simulink model "cplxfir"  (Simulink 7.4)
settings: Solver=VariableStepDiscrete  SolverMode=SingleTasking  StartTime=0.0  StopTime=.01  FixedStep=1/Fs  RelTol=1e-3
PreLoadFcn:
  | cplxfir_PreLoadFcn
values from neighbouring files (symbols this model uses):
  coefwidth = 14    [cplxfir_PreLoadFcn.m]
  Fs = 1000000    [cmplx_coef.mat]
  im_num = [0 0.000398348009628 0.00104175614283 0.00211081091276 0.00279070112666 0.00258044261419 0.000985988872345 -0.0017034426046 -0.00446098448822 -0.00593463418221 -0.00527808120455 -0.00289469541568 ... (64 elements, 1x64)]    [cmplx_coef.mat]
  re_num = [0.000255022274952 0.000745256708112 0.000696079200562 0.00020789672902 -0.00115594625519 -0.00314427842297 -0.00495690079674 -0.00561549770163 -0.00446098448822 -0.0018002515976 0.00104987562762 0.00237561513355 ... (64 elements, 1x64)]    [cmplx_coef.mat]
undefined symbols (not defined in the file or in its folder): c, C, D, d, j, sided, Two, xlipgetpartsetting
libraries: xbsIndex_r4 x23, dsparch3 x4, dspsnks4 x3, dspobslib x2, dspsrcs4 x1, xbsCopyrightNotice_r4 x1
settings Model: Creator=mklusman  LastModifiedBy=douangp
settings DataIOCC: SignalLoggingName=sigsOut
settings OptimizationCC: BooleanDataType=off  InitFltsAndDblsToZero=on
settings DebuggingCC: SaveWithParameterizedLinksMsg=none  SignalResolutionControl=TryResolveAllWithWarning  SolverPrmCheckMsg=none  MultiTaskDSMMsg=warning  MultiTaskCondExecSysMsg=none  StrictBusMsg=None
settings HardwareCC: TargetUnknown=on
settings RTWCC: IncludeERTFirstTime=on
settings GRTTargetCC: TargetFcnLib=ansi_tfl_tmw.mat

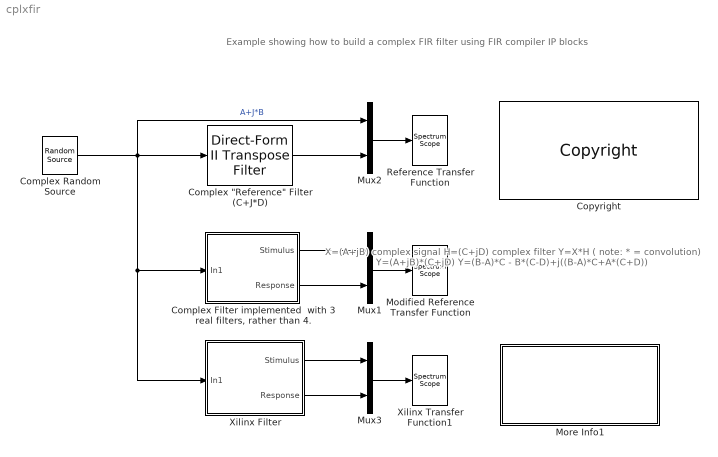
== system cplxfir ==
  note: X=(A+jB)     complex signal
      | H=(C+jD)     complex filter
      | Y=X*H ( note: * = convolution)
      | Y=(A+jB)*(C+jD)
      | Y=(B-A)*C - B*(C-D)+j((B-A)*C+A*(C+D))
  note: Example showing how to build a complex FIR filter
      |  using FIR compiler IP blocks
  "Complex \"Reference\" Filter (C+J*D)" : dsparch3/Direct-Form II Transpose Filter  num=[re_num+j*im_num]  den=1  ic=0
  "Complex Filter implemented  with 3 real filters, rather than 4.  " : Subsystem
  Complex Random Source : dspsrcs4/Random Source  SrcType=Uniform  NormMethod=Ziggurat  CltLength=12  MinVal=-.99  MaxVal=0.99  MeanVal=0  VarVal=1  RepMode=Not repeatable  rawSeed=1  IsInherit=off  SampMode=Discrete  SampTime=1/Fs  SampFrame=1  DataType=Double  OutComplex=Complex
  Copyright : xbsCopyrightNotice_r4/Copyright  copyrighttext="Copyright (c) 2010  by  Xilinx, Inc. All rights reserved.<br><br>This file contains proprietary, confidential information of Xilinx, Inc., is distributed under licensefrom Xilinx, Inc., and may be used, copied and/or disclosed only pursuant to the terms of a valid licenseagreement with Xilinx, Inc. Xilinx hereby grants you a license to use this file solely for design,simulation, implementation and creation of design files limited to Xilinx devices or technologies. Use with non-Xilinx devices or technologies is expressly prohibited and immediately terminates your license unless covered by a separate agreement.<br><br>Xilinx is providing this design, code, or information \"as-is\" solely for use in developing programs and solutions for Xilinx devices, with no obligation on the part of Xilinx to provide support. By providingthis design, code, or information as one possible implementation of this feature, application or standard,Xilinx is making no representation that this implementation is free from any claims of infringement. Youare responsible for obtaining any rights you may require for your implementation. Xilinx expressly disclaimsany warranty whatsoever with respect to the adequacy of the implementation, including but not limited to anywarranties or representations that this implementation is free from claims of infringement, implied warrantiesof merchantability or fitness for a particular purpose.<br><br>Xilinx products are not intended for use in life support appliances, devices, or systems. Use in such applications is expressly prohibited.<br><br>Any modifications that are made to the Source Code are done at the user's sole risk and will be unsupported.<br><br>This copyright and support notice must be retained as part of this text at all times. (c) Copyright 1995-2010 Xilinx, Inc. All rights reserved."  block_type=copyright
      settings: block_version=10.1.3
      settings: infoedit=|
      | Copyright(C) 2008 by  Xilinx, Inc. All rights reserved.<br>
      | <br>
      | This file contains proprietary, confidential information of Xilinx, Inc., is distributed under license
      | from Xilinx, Inc., and may be used, copied and/or disclosed only pursuant to the terms of a valid license
      | agreement with Xilinx, Inc. Xilinx hereby grants you a license to use this file solely for design,
      | simulation, implementation and creation of design files limited to Xilinx devices or technologies. Use
      | with non-Xilinx devices or technologies is expressly prohibited and immediately terminates your license
      | unless covered by a separate agreement.<br>
      | <br>
      | Xilinx is providing this design, code, or information "as-is" solely for use in developing programs and
      | solutions for Xilinx devices, with no obligation on the part of Xilinx to provide support. By providing
      | this design, code, or information as one possible implementation of this feature, application or standard,
      | Xilinx is making no representation that this implementation is free from any claims of infringement. You
      | are responsible for obtaining any rights you may require for your implementation. Xilinx expressly disclaims
      | any warranty whatsoever with respect to the adequacy of the implementation, including but not limited to any
      | warranties or representations that this implementation is free from claims of infringement, implied warranties
      | of merchantability or fitness for a particular purpose.<br>
      | <br>
      | Xilinx products are not intended for use in life support appliances, devices, or systems. Use in such
      | applications is expressly prohibited.<br>
      | <br>
      | Any modifications that are made to the Source Code are done at the user's sole risk and will be unsupported.<br>
      | <br>
      | This copyright and support notice must be retained as part of this text at all times.
      | (c) Copyright 1995-2008 Xilinx, Inc. All rights reserved.
  Modified Reference Transfer Function : dspsnks4/Spectrum Scope  DialogController=dspdialog.SpectrumScope  DialogControllerArgs=DataTag1  SystemSampleTime=-1  ScopeProperties=off  Domain=Frequency  HorizSpan=1  UseBuffer=on  BufferSize=512  Overlap=64  inpFftLenInherit=off  FFTlength=512  numAvg=2  DisplayProperties=off  AxisGrid=on  Memory=off  FrameNumber=on  AxisLegend=on  AxisZoom=off  OpenScopeAtSimStart=on  OpenScopeImmediately=off  FigPos=[-999 166 385 234]  AxisProperties=on  XUnits=Hertz  XRange=Two-sided ((-Fs/2...Fs/2])  XDisplay=0  InheritXIncr=on  XIncr=1.0  XLabel=Samples  XLimit=User-defined  YUnits=dBm  XMax=500000  XMin=0  YLabel=Magnitude, dB  LineProperties=off  LineColors=[0 0 1]|[1 0 0]  wintypeSpecScope=Hann  RsSpecScope=50  betaSpecScope=5  winsampSpecScope=Periodic  XAxisParamsVer=6.9
      settings: YMin=-91.486  YMax=10.5651
  More Info1 : Subsystem
      mask Display: disp('Double click\n for\n more information.')
  Mux1 : Mux  Inputs=2
  Mux2 : Mux  Inputs=2
  Mux3 : Mux  Inputs=2
  Reference Transfer Function : dspsnks4/Spectrum Scope  DialogController=dspdialog.SpectrumScope  DialogControllerArgs=DataTag2  SystemSampleTime=-1  ScopeProperties=off  Domain=Frequency  HorizSpan=1  UseBuffer=on  BufferSize=512  Overlap=64  inpFftLenInherit=off  FFTlength=512  numAvg=2  DisplayProperties=off  AxisGrid=on  Memory=off  FrameNumber=on  AxisLegend=on  AxisZoom=off  OpenScopeAtSimStart=on  OpenScopeImmediately=off  FigPos=[-993 480 377 230]  AxisProperties=on  XUnits=Hertz  XRange=Two-sided ((-Fs/2...Fs/2])  XDisplay=0  InheritXIncr=on  XIncr=1.0  XLabel=Samples  XLimit=User-defined  YUnits=dBm  XMax=500000  XMin=0  YLabel=Magnitude, dB  LineProperties=off  LineColors=[0 0 1]|[1 0 0]  wintypeSpecScope=Hann  RsSpecScope=50  betaSpecScope=5  winsampSpecScope=Periodic  XAxisParamsVer=6.9
      settings: YMin=-91.486  YMax=10.5651
  Xilinx Transfer Function1 : dspsnks4/Spectrum Scope  DialogController=dspdialog.SpectrumScope  DialogControllerArgs=DataTag3  SystemSampleTime=-1  ScopeProperties=off  Domain=Frequency  HorizSpan=1  UseBuffer=on  BufferSize=512  Overlap=64  inpFftLenInherit=off  FFTlength=512  numAvg=2  DisplayProperties=off  AxisGrid=on  Memory=off  FrameNumber=on  AxisLegend=on  AxisZoom=off  OpenScopeAtSimStart=on  OpenScopeImmediately=off  FigPos=[-611 244 385 234]  AxisProperties=on  XUnits=Hertz  XRange=Two-sided ((-Fs/2...Fs/2])  XDisplay=0  InheritXIncr=on  XIncr=1.0  XLabel=Samples  XLimit=User-defined  YUnits=dBm  XMax=500000  XMin=0  YLabel=Magnitude, dB  LineProperties=off  LineColors=[0 0 1]|[1 0 0]  wintypeSpecScope=Hann  RsSpecScope=50  betaSpecScope=5  winsampSpecScope=Periodic  XAxisParamsVer=6.9
      settings: YMin=-86.1357  YMax=10.4347
  Xilinx Filter : Subsystem
  wires:
  Complex Random Source/1 -> "Complex \"Reference\" Filter (C+J*D)"/1, Xilinx Filter/1(In1), "Complex Filter implemented  with 3 real filters, rather than 4.  "/1(In1), Mux2/1  "A+J*B"
  Xilinx Filter/2("Response ") -> Mux3/2
  "Complex \"Reference\" Filter (C+J*D)"/1 -> Mux2/2
  "Complex Filter implemented  with 3 real filters, rather than 4.  "/2(Response) -> Mux1/2
  Xilinx Filter/1("Stimulus ") -> Mux3/1
  Mux3/1 -> Xilinx Transfer Function1/1
  "Complex Filter implemented  with 3 real filters, rather than 4.  "/1(Stimulus) -> Mux1/1
  Mux1/1 -> Modified Reference Transfer Function/1
  Mux2/1 -> Reference Transfer Function/1

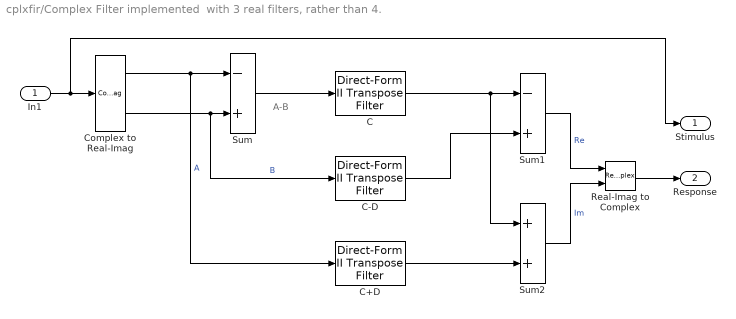
== system cplxfir/Complex Filter implemented  with 3 real filters, rather than 4.   ==
  note: A-B
  In1 : Inport  OutDataType=sfix(16)  OutScaling=2^0
  C : dsparch3/Direct-Form II Transpose Filter  num="[re_num]   %    c"  den=1  ic=0
  C+D : dsparch3/Direct-Form II Transpose Filter  num="[re_num+im_num]  % C+D"  den=1  ic=0
  C-D : dsparch3/Direct-Form II Transpose Filter  num="[re_num-im_num]    % c-d"  den=1  ic=0
  Complex to Real-Imag : ComplexToRealImag
  Real-Imag to Complex : RealImagToComplex
  Sum : Sum  Inputs=-+  OutDataType=sfix(16)  OutScaling=2^0  SaturateOnIntegerOverflow=on  InputSameDT=on  OutDataTypeStr=Inherit: Same as first input
  Sum1 : Sum  Inputs=-+  OutDataType=sfix(16)  OutScaling=2^0  SaturateOnIntegerOverflow=on  InputSameDT=on  OutDataTypeStr=Inherit: Same as first input
  Sum2 : Sum  OutDataType=sfix(16)  OutScaling=2^0  SaturateOnIntegerOverflow=on  InputSameDT=on  OutDataTypeStr=Inherit: Same as first input
  Stimulus : Outport  OutDataType=sfix(16)  OutScaling=2^0
  Response : Outport  Port=2  OutDataType=sfix(16)  OutScaling=2^0
  wires:
  Complex to Real-Imag/1 -> Sum/1, C+D/1  "A"
  Complex to Real-Imag/2 -> Sum/2, C-D/1  "B"
  Sum/1 -> C/1
  C/1 -> Sum1/1, Sum2/1
  C-D/1 -> Sum1/2
  C+D/1 -> Sum2/2
  Sum1/1 -> Real-Imag to Complex/1  "Re"
  Sum2/1 -> Real-Imag to Complex/2  "Im"
  In1/1 -> Complex to Real-Imag/1, Stimulus/1
  Real-Imag to Complex/1 -> Response/1

== system cplxfir/More Info1 ==
  note: This design shows how to migrate a complex filter design from using DAFIR to FIR
      | Compiler. The model was originally constructed using DAFIR as provided
      | by System Generator design example.   The migration process is seamless and
      | straight forward.
      |
      | The "cplxfir_PreLoadFcn.m" file is preloaded when opening the model. It also loads
      | filter coefficients stored in "cmplx_coef.mat" file. Out of the box, the model can be
      | simulated and compared between Xilinx transfer function, simulation results and
      | two other models.
      |
      | The following quality of results (QoR) are used as a reference, baseline only and they may be
      | varied within an acceptable range from one release to the next.
      | This design occupies 274 Slice LUTs, 486 Slice Registers, and 192 dedicated multipliers of
      | a Xilinx xc6vsx315t-1 part and operates close to 350 MHz (11.2 software, VHDL synthesized with
      | XST). The QoR may be further improved in both area utilizations and speed.
  note: Example showing how to build a complex FIR filter
      |  using FIR compiler IP blocks

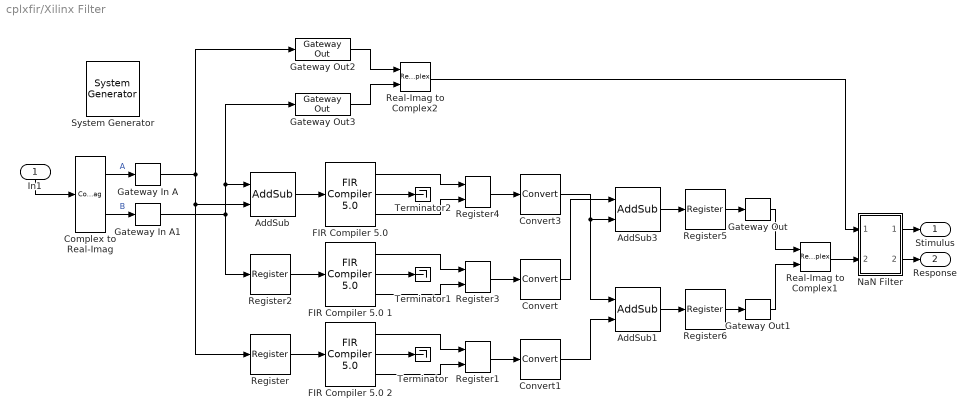
== system cplxfir/Xilinx Filter ==
  In1 : Inport  OutDataType=sfix(16)  OutScaling=2^0
  " System Generator" : xbsIndex_r4/ System Generator  Tag=genX  SystemSampleTime=-1  xilinxfamily=virtex6  part=xc6vsx315t  speed=-1  package=ff1156  synthesis_tool=XST  clock_wrapper=Clock Enables  directory=./timing  testbench=off  simulink_period=1/1000000  sysclk_period=10  dcm_input_clock_period=5  incr_netlist=off  trim_vbits=According to Block Masks  dbl_ovrd=According to Block Masks  core_generation=According to Block Masks  run_coregen=off  deprecated_control=off  eval_field=0  block_type=sysgen
      settings: block_version=9.1.01
  AddSub : xbsIndex_r4/AddSub  mode=Subtraction  use_carryin=off  use_carryout=off  en=off  latency=1  precision=Full  arith_type=Unsigned  n_bits=8  bin_pt=2  quantization=Truncate  overflow=Wrap  dbl_ovrd=off  use_behavioral_HDL=on  hw_selection=Fabric  pipelined=off  use_rpm=off  block_type=addsub
      settings: xl_area=[0, 0, 0, 0, 0, 0, 0]  block_version=VER_STRING_GOES_HERE
  AddSub1 : xbsIndex_r4/AddSub  mode=Addition  use_carryin=off  use_carryout=off  en=off  latency=1  precision=Full  arith_type=Unsigned  n_bits=8  bin_pt=2  quantization=Truncate  overflow=Wrap  dbl_ovrd=off  use_behavioral_HDL=on  hw_selection=Fabric  pipelined=off  use_rpm=off  block_type=addsub
      settings: xl_area=[0, 0, 0, 0, 0, 0, 0]  block_version=VER_STRING_GOES_HERE
  AddSub3 : xbsIndex_r4/AddSub  mode=Subtraction  use_carryin=off  use_carryout=off  en=off  latency=1  precision=Full  arith_type=Unsigned  n_bits=8  bin_pt=2  quantization=Truncate  overflow=Wrap  dbl_ovrd=off  use_behavioral_HDL=on  hw_selection=Fabric  pipelined=off  use_rpm=off  block_type=addsub
      settings: xl_area=[0, 0, 0, 0, 0, 0, 0]  block_version=VER_STRING_GOES_HERE
  Complex to Real-Imag : ComplexToRealImag
  Convert : xbsIndex_r4/Convert  arith_type="Signed  (2's comp)"  n_bits=coefwidth  bin_pt=coefwidth-2  quantization=Truncate  overflow=Wrap  en=off  latency=0  dbl_ovrd=off  pipeline=off  block_type=convert
      settings: infoedit=The input is presented at the output after quantization and overflow effects.<P><P>Hardware notes: Additional hardware is used when rounding or saturation is selected and output width is less than the input width.  xl_area=[0, 0, 0, 0, 0, 0, 0]  block_version=VER_STRING_GOES_HERE
  Convert1 : xbsIndex_r4/Convert  arith_type="Signed  (2's comp)"  n_bits=coefwidth  bin_pt=coefwidth-2  quantization=Truncate  overflow=Wrap  en=off  latency=0  dbl_ovrd=off  pipeline=off  block_type=convert
      settings: infoedit=The input is presented at the output after quantization and overflow effects.<P><P>Hardware notes: Additional hardware is used when rounding or saturation is selected and output width is less than the input width.  xl_area=[0, 0, 0, 0, 0, 0, 0]  block_version=VER_STRING_GOES_HERE
  Convert3 : xbsIndex_r4/Convert  arith_type="Signed  (2's comp)"  n_bits=coefwidth  bin_pt=coefwidth-2  quantization=Truncate  overflow=Wrap  en=off  latency=0  dbl_ovrd=off  pipeline=off  block_type=convert
      settings: infoedit=The input is presented at the output after quantization and overflow effects.<P><P>Hardware notes: Additional hardware is used when rounding or saturation is selected and output width is less than the input width.  xl_area=[0, 0, 0, 0, 0, 0, 0]  block_version=VER_STRING_GOES_HERE
  "FIR Compiler 5.0 " : xbsIndex_r4/FIR Compiler 5.0   coefficientvector=re_num  coefficient_sets=1  filter_type=Single_Rate  rate_change_type=Integer  interpolation_rate=1  decimation_rate=1  zero_pack_factor=1  number_channels=1  ratespecification=Maximum_Possible  sampleperiod=1  hardwareoversamplingrate=1  filter_architecture=Transpose_Multiply_Accumulate  coefficient_reload=off  coefficient_structure=Non_Symmetric  coefficient_sign=Signed  quantization=Quantize_Only  coefficient_width=14  bestprecision=on  coefficient_fractional_bits=6  number_paths=1  output_rounding_mode=Full_Precision  output_width=30  allow_rounding_approximation=off  optimization_goal=Speed  has_sclr=off  has_data_valid=off  has_nd=off  has_ce=off  usechan_in_adv=off  chan_in_adv=0  data_buffer_type=Automatic  coefficient_buffer_type=Automatic  input_buffer_type=Automatic  output_buffer_type=Automatic  preference_for_other_storage=Automatic  multi_column_support=Disabled  columnconfig='1'  inter_column_pipe_length=4  passband_min=0.0  passband_max=0.5  stopband_min=0.5  stopband_max=1.0  filter_selection=1  gui_behaviour=Sysgen  registered_output=true  data_sign=Signed  data_width=16  wrapper_available=true  ip_wrap_arbitrary_binary_point=true  ip_name=FIR Compiler  ip_version=5.0  dsptool_ready=true  ipcore_usecache=true  ipcore_useipmodelcache=true  ipcore_xco_need_fpga_part=true  port_translation_map={ 'ce' => 'en', 'sclr' => 'rst' }  run_core_at_system_period=true  ipcore_fpga_part=xlipgetpartsetting(gcb, {'virtex4', 'xc4vsx35', '-10', 'ff668'})  structural_sim=false  block_type=fir_compiler_v5_0
      settings: block_version=11.2
  FIR Compiler 5.0 1 : xbsIndex_r4/FIR Compiler 5.0   coefficientvector=re_num  coefficient_sets=1  filter_type=Single_Rate  rate_change_type=Integer  interpolation_rate=1  decimation_rate=1  zero_pack_factor=1  number_channels=1  ratespecification=Maximum_Possible  sampleperiod=1  hardwareoversamplingrate=1  filter_architecture=Transpose_Multiply_Accumulate  coefficient_reload=off  coefficient_structure=Non_Symmetric  coefficient_sign=Signed  quantization=Quantize_Only  coefficient_width=14  bestprecision=on  coefficient_fractional_bits=6  number_paths=1  output_rounding_mode=Full_Precision  output_width=30  allow_rounding_approximation=off  optimization_goal=Speed  has_sclr=off  has_data_valid=off  has_nd=off  has_ce=off  usechan_in_adv=off  chan_in_adv=0  data_buffer_type=Automatic  coefficient_buffer_type=Automatic  input_buffer_type=Automatic  output_buffer_type=Automatic  preference_for_other_storage=Automatic  multi_column_support=Disabled  columnconfig='1'  inter_column_pipe_length=4  passband_min=0.0  passband_max=0.5  stopband_min=0.5  stopband_max=1.0  filter_selection=1  gui_behaviour=Sysgen  registered_output=true  data_sign=Signed  data_width=16  wrapper_available=true  ip_wrap_arbitrary_binary_point=true  ip_name=FIR Compiler  ip_version=5.0  dsptool_ready=true  ipcore_usecache=true  ipcore_useipmodelcache=true  ipcore_xco_need_fpga_part=true  port_translation_map={ 'ce' => 'en', 'sclr' => 'rst' }  run_core_at_system_period=true  ipcore_fpga_part=xlipgetpartsetting(gcb, {'virtex4', 'xc4vsx35', '-10', 'ff668'})  structural_sim=false  block_type=fir_compiler_v5_0
      settings: block_version=11.2
  FIR Compiler 5.0 2 : xbsIndex_r4/FIR Compiler 5.0   coefficientvector=re_num  coefficient_sets=1  filter_type=Single_Rate  rate_change_type=Integer  interpolation_rate=1  decimation_rate=1  zero_pack_factor=1  number_channels=1  ratespecification=Maximum_Possible  sampleperiod=1  hardwareoversamplingrate=1  filter_architecture=Transpose_Multiply_Accumulate  coefficient_reload=off  coefficient_structure=Non_Symmetric  coefficient_sign=Signed  quantization=Quantize_Only  coefficient_width=14  bestprecision=on  coefficient_fractional_bits=6  number_paths=1  output_rounding_mode=Full_Precision  output_width=30  allow_rounding_approximation=off  optimization_goal=Speed  has_sclr=off  has_data_valid=off  has_nd=off  has_ce=off  usechan_in_adv=off  chan_in_adv=0  data_buffer_type=Automatic  coefficient_buffer_type=Automatic  input_buffer_type=Automatic  output_buffer_type=Automatic  preference_for_other_storage=Automatic  multi_column_support=Disabled  columnconfig='1'  inter_column_pipe_length=4  passband_min=0.0  passband_max=0.5  stopband_min=0.5  stopband_max=1.0  filter_selection=1  gui_behaviour=Sysgen  registered_output=true  data_sign=Signed  data_width=16  wrapper_available=true  ip_wrap_arbitrary_binary_point=true  ip_name=FIR Compiler  ip_version=5.0  dsptool_ready=true  ipcore_usecache=true  ipcore_useipmodelcache=true  ipcore_xco_need_fpga_part=true  port_translation_map={ 'ce' => 'en', 'sclr' => 'rst' }  run_core_at_system_period=true  ipcore_fpga_part=xlipgetpartsetting(gcb, {'virtex4', 'xc4vsx35', '-10', 'ff668'})  structural_sim=false  block_type=fir_compiler_v5_0
      settings: block_version=11.2
  Gateway In A : xbsIndex_r4/Gateway In  arith_type="Signed  (2's comp)"  n_bits=coefwidth  bin_pt=coefwidth-2  quantization="Round  (unbiased: +/- Inf)"  overflow=Saturate  period=1/Fs  dbl_ovrd=off  timing_constraint=None  locs_specified=off  LOCs={}  hdl_port=on  block_type=gatewayin
      settings: infoedit="Gateway in block.  Converts inputs of type Simulink integer, double and fixed point to  Xilinx fixed point type.<P><P>Hardware notes:  In hardware these blocks become top level input ports."  xl_area=[0, 0, 0, 0, 0, 0, 0]  block_version=VER_STRING_GOES_HERE
  Gateway In A1 : xbsIndex_r4/Gateway In  arith_type="Signed  (2's comp)"  n_bits=coefwidth  bin_pt=coefwidth-2  quantization="Round  (unbiased: +/- Inf)"  overflow=Saturate  period=1/Fs  dbl_ovrd=off  timing_constraint=None  locs_specified=off  LOCs={}  hdl_port=on  block_type=gatewayin
      settings: infoedit="Gateway in block.  Converts inputs of type Simulink integer, double and fixed point to  Xilinx fixed point type.<P><P>Hardware notes:  In hardware these blocks become top level input ports."  xl_area=[0, 0, 0, 0, 0, 0, 0]  block_version=VER_STRING_GOES_HERE
  Gateway Out : xbsIndex_r4/Gateway Out  hdl_port=on  timing_constraint=None  locs_specified=off  LOCs={}  block_type=gatewayout
      settings: infoedit="Gateway out block.  Converts Xilinx fixed point inputs into ouputs of type Simulink integer, double, or fixed point.<P><P>Hardware notes:  In hardware these blocks become top level output ports or are discarded, depending on how they are configured."  xl_area=[0, 0, 0, 0, 0, 0, 0]  block_version=VER_STRING_GOES_HERE
  Gateway Out1 : xbsIndex_r4/Gateway Out  hdl_port=on  timing_constraint=None  locs_specified=off  LOCs={}  block_type=gatewayout
      settings: infoedit="Gateway out block.  Converts Xilinx fixed point inputs into ouputs of type Simulink integer, double, or fixed point.<P><P>Hardware notes:  In hardware these blocks become top level output ports or are discarded, depending on how they are configured."  xl_area=[0, 0, 0, 0, 0, 0, 0]  block_version=VER_STRING_GOES_HERE
  Gateway Out2 : xbsIndex_r4/Gateway Out  hdl_port=off  timing_constraint=None  locs_specified=off  LOCs={}  block_type=gatewayout
      settings: infoedit="Gateway out block.  Converts Xilinx fixed point inputs into ouputs of type Simulink integer, double, or fixed point.<P><P>Hardware notes:  In hardware these blocks become top level output ports or are discarded, depending on how they are configured."  xl_area=[0, 0, 0, 0, 0, 0, 0]  block_version=VER_STRING_GOES_HERE
  Gateway Out3 : xbsIndex_r4/Gateway Out  hdl_port=off  timing_constraint=None  locs_specified=off  LOCs={}  block_type=gatewayout
      settings: infoedit="Gateway out block.  Converts Xilinx fixed point inputs into ouputs of type Simulink integer, double, or fixed point.<P><P>Hardware notes:  In hardware these blocks become top level output ports or are discarded, depending on how they are configured."  xl_area=[0, 0, 0, 0, 0, 0, 0]  block_version=VER_STRING_GOES_HERE
  NaN Filter : Subsystem
  Real-Imag to Complex1 : RealImagToComplex
  Real-Imag to Complex2 : RealImagToComplex
  Register{,2,5..6} (4 alike) : xbsIndex_r4/Register  init=0  rst=off  en=off  dbl_ovrd=off  block_type=register
      settings: xl_area=[0, 0, 0, 0, 0, 0, 0]  block_version=VER_STRING_GOES_HERE
  Register1 : xbsIndex_r4/Register  init=0  rst=off  en=on  dbl_ovrd=off  block_type=register
  Register3 : xbsIndex_r4/Register  init=0  rst=off  en=on  dbl_ovrd=off  block_type=register
  Register4 : xbsIndex_r4/Register  init=0  rst=off  en=on  dbl_ovrd=off  block_type=register
  Terminator : Terminator
  Terminator1 : Terminator
  Terminator2 : Terminator
  "Stimulus " : Outport  OutDataType=sfix(16)  OutScaling=2^0
  "Response " : Outport  Port=2  OutDataType=sfix(16)  OutScaling=2^0
  wires:
  Complex to Real-Imag/2 -> Gateway In A1/1  "B"
  Complex to Real-Imag/1 -> Gateway In A/1  "A"
  Gateway In A/1 -> AddSub/2, Register/1, Gateway Out2/1
  Gateway In A1/1 -> Gateway Out3/1, AddSub/1, Register2/1
  Register/1 -> FIR Compiler 5.0 2/1
  AddSub3/1 -> Register5/1
  AddSub1/1 -> Register6/1
  Gateway Out/1 -> Real-Imag to Complex1/1
  Gateway Out1/1 -> Real-Imag to Complex1/2
  In1/1 -> Complex to Real-Imag/1
  Gateway Out3/1 -> Real-Imag to Complex2/2
  Gateway Out2/1 -> Real-Imag to Complex2/1
  Convert3/1 -> AddSub3/2, AddSub1/1
  Convert/1 -> AddSub3/1
  Convert1/1 -> AddSub1/2
  Real-Imag to Complex1/1 -> NaN Filter/2(In2)
  NaN Filter/2(Out2) -> "Response "/1
  NaN Filter/1(Out1) -> "Stimulus "/1
  Real-Imag to Complex2/1 -> NaN Filter/1(In1)
  FIR Compiler 5.0 2/2 -> Terminator/1
  FIR Compiler 5.0 2/1 -> Register1/1
  FIR Compiler 5.0 2/3 -> Register1/2
  FIR Compiler 5.0 1/1 -> Register3/1
  FIR Compiler 5.0 1/3 -> Register3/2
  FIR Compiler 5.0 1/2 -> Terminator1/1
  Register2/1 -> FIR Compiler 5.0 1/1
  Register3/1 -> Convert/1
  Register1/1 -> Convert1/1
  "FIR Compiler 5.0 "/3 -> Register4/2
  "FIR Compiler 5.0 "/2 -> Terminator2/1
  AddSub/1 -> "FIR Compiler 5.0 "/1
  Register4/1 -> Convert3/1
  Register5/1 -> Gateway Out/1
  Register6/1 -> Gateway Out1/1
  "FIR Compiler 5.0 "/1 -> Register4/1

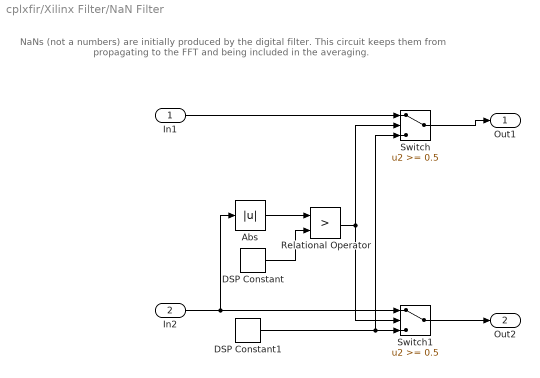
== system cplxfir/Xilinx Filter/NaN Filter ==
  note: NaNs  (not a numbers) are initially produced by the digital filter.
      | This circuit keeps them from propagating to the FFT and being
      | included in the averaging.
  In1 : Inport  OutDataType=sfix(16)  OutScaling=2^0
  In2 : Inport  Port=2  OutDataType=sfix(16)  OutScaling=2^0
  Abs : Abs  SaturateOnIntegerOverflow=on
  DSP Constant : dspobslib/DSP Constant  SystemSampleTime=-1  Value=-inf  SampleMode=Discrete  discreteOutput=Sample-based  continuousOutput=Sample-based  sampTime=1/Fs  framePeriod=1/Fs  dataType=Inherit from 'Constant value'  isSigned=on  wordLen=16  udDataType=sfix(16)  fracBitsMode=Best precision  numFracBits=15  InterpretAs1D=off  Ts=1/Fs  FramebasedOutput=off
  DSP Constant1 : dspobslib/DSP Constant  SystemSampleTime=-1  Value=0+j*eps  SampleMode=Discrete  discreteOutput=Sample-based  continuousOutput=Sample-based  sampTime=1/Fs  framePeriod=1/Fs  dataType=Inherit from 'Constant value'  isSigned=on  wordLen=16  udDataType=sfix(16)  fracBitsMode=Best precision  numFracBits=15  InterpretAs1D=off  Ts=1/Fs  FramebasedOutput=off
  Relational Operator : RelationalOperator  Operator=>  InputSameDT=on
  Switch : Switch  Threshold=0.5  SaturateOnIntegerOverflow=on  InputSameDT=on
  Switch1 : Switch  Threshold=0.5  SaturateOnIntegerOverflow=on  InputSameDT=on
  Out1 : Outport  OutDataType=sfix(16)  OutScaling=2^0
  Out2 : Outport  Port=2  OutDataType=sfix(16)  OutScaling=2^0
  wires:
  DSP Constant1/1 -> Switch/3, Switch1/3
  Relational Operator/1 -> Switch1/2, Switch/2
  DSP Constant/1 -> Relational Operator/2
  Abs/1 -> Relational Operator/1
  Switch1/1 -> Out2/1
  Switch/1 -> Out1/1
  In1/1 -> Switch/1
  In2/1 -> Abs/1, Switch1/1
